simulink model "untitled"  (R2018b)
settings: Solver=VariableStepAuto  StartTime=0.0  StopTime=0  RelTol=1e-3
libraries: commrandsrc3 x1
settings Model: Creator=DSP_26  LastModifiedBy=DSP_26

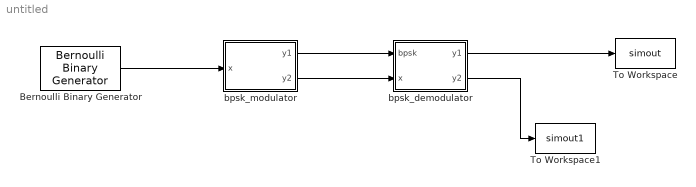
== system untitled ==
  Bernoulli Binary Generator : commrandsrc3/Bernoulli Binary Generator  ProbabilityOfZero=0.5  SeedSource=Auto  Seed=0  SampleTime=1  SamplesPerFrame=10000  OutputDataType=double  SimulateUsing=Interpreted execution
  To Workspace : ToWorkspace  VariableName=simout  SampleTime=-1
      settings: Save2DSignal=2-D array (concatenate along first dimension)
  To Workspace1 : ToWorkspace  VariableName=simout1  SampleTime=-1
      settings: Save2DSignal=2-D array (concatenate along first dimension)
  bpsk_demodulator : MATLAB Function  TreatAsAtomicUnit=on
  bpsk_modulator : MATLAB Function  TreatAsAtomicUnit=on
  wires:
  Bernoulli Binary Generator/1 -> bpsk_modulator/1(x)
  bpsk_modulator/1(y1) -> bpsk_demodulator/1(bpsk)
  bpsk_demodulator/1(y1) -> To Workspace/1
  bpsk_demodulator/2(y2) -> To Workspace1/1
  bpsk_modulator/2(y2) -> bpsk_demodulator/2(x)

== matlab function untitled/bpsk_demodulator ==
  data: bpsk input; y1 output; y2 output; x input
function [y1,y2] = bpsk_demodulator(bpsk,x)

snrd = zeros(1,7);
a = 0;
for r=1:7
    snrd(r) = a;
    a = a+4;
end

sigma = zeros(1,7);
snrl = zeros(1,7);
perror = zeros(1,7);
terror = zeros(1,7);
bpsk1 = zeros(1,10000);

for r=1:7
    h = randn(1,10000) + 1j*randn(1,10000);
    noise = randn(1,10000) + 1j*randn(1,10000);
    snrl(r) = 10^(snrd(r)/10);
    sigma(r) = sqrt(10.^(-snrl(r)/10));
    y = h.*bpsk + noise*sigma(r);
    y = y./h;
    for n=1:10000
        if(real(y(n))>0)
            bpsk1(n) = 1;
        else
            bpsk1(n) = 0;
        end
    end
    perror(r) = mean(abs(x-bpsk1));
    %perror(r) = sum(abs((x-bpsk1)/2))/10000;
    terror(r) = 0.5*(1-sqrt(snrl(r)/(2+snrl(r))));
end

y1 = perror;
y2 = terror;

== matlab function untitled/bpsk_modulator ==
  data: x input; y1 output; y2 output
function [y1,y2] = bpsk_modulator(x)
x = transpose(x);
bpsk = zeros(1,10000);
for n=1:10000
    if(x(n)==0)
        bpsk(n) = -1;
    else
        bpsk(n) = 1;
    end
end
y1 = bpsk;
y2 = x;
